simulink model "N_scheme_RP4_U"  (R2024b)
settings: Solver=VariableStepAuto  StartTime=0.0  StopTime=10.0  RelTol=1e-3
values from neighbouring files (symbols this model uses):
  Ga = -12500    [p23.m]
  Gf = 1/(Kd*Gs)    (= 0.25)    [p23.m]
  Gs = 2    [p23.m]
libraries: cstblocks x4
settings Model: Creator=adrian  LastModifiedBy=adrian

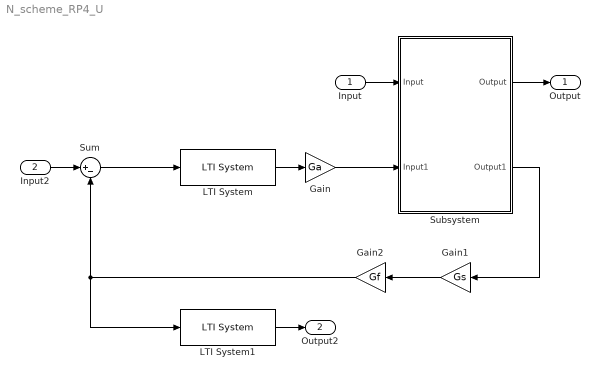
== system N_scheme_RP4_U ==
  Input : Inport
  Input2 : Inport  Port=2
  Gain : Gain  Gain=Ga
  Gain1 : Gain  Gain=Gs
  Gain2 : Gain  Gain=Gf
  LTI System : cstblocks/LTI System  sys=Gc  IC=[]  PadeOrder=0
  LTI System1 : cstblocks/LTI System  sys=WT_mu_RP4  IC=[]  PadeOrder=0
  Subsystem : Subsystem
  Sum : Sum  Inputs=|+-
  Output : Outport
  Output2 : Outport  Port=2
  wires:
  Gain/1 -> Subsystem/2(Input1)
  Input/1 -> Subsystem/1(Input)
  LTI System/1 -> Gain/1
  Subsystem/2(Output1) -> Gain1/1
  Subsystem/1(Output) -> Output/1
  Gain1/1 -> Gain2/1
  Gain2/1 -> Sum/2, LTI System1/1
  Sum/1 -> LTI System/1
  Input2/1 -> Sum/1
  LTI System1/1 -> Output2/1

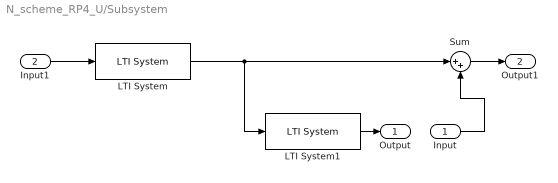
== system N_scheme_RP4_U/Subsystem ==
  Input : Inport
  Input1 : Inport  Port=2
  LTI System : cstblocks/LTI System  sys=Gpn  IC=[]  PadeOrder=0
  LTI System1 : cstblocks/LTI System  sys=Wu  IC=[]  PadeOrder=0
  Sum : Sum  Inputs=|++
  Output : Outport
  Output1 : Outport  Port=2
  wires:
  LTI System/1 -> LTI System1/1, Sum/1
  LTI System1/1 -> Output/1
  Input/1 -> Sum/2
  Sum/1 -> Output1/1
  Input1/1 -> LTI System/1
